simulink model "transistor_switch_1"  (Simulink 7.4)
settings: Solver=ode23s  StartTime=0.0  StopTime=200e-6  MaxStep=10e-9  RelTol=1e-4
libraries: powerlib x7, simpower_extensions_1 x1
settings Model: Creator=Dick  LastModifiedBy=Dick

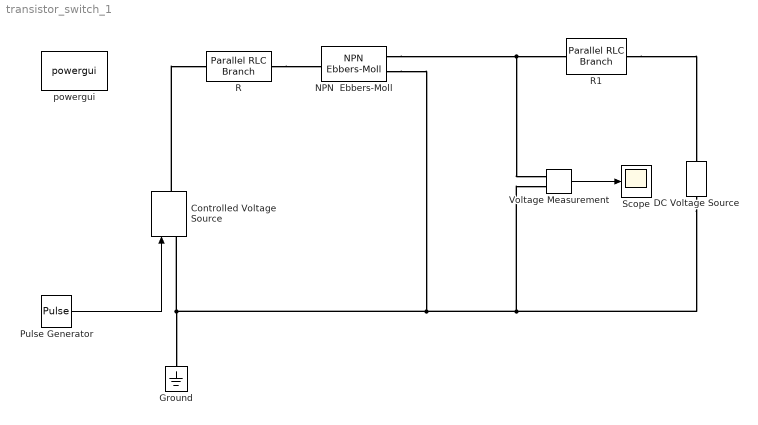
== system transistor_switch_1 ==
  " R" : powerlib/Elements/Parallel RLC Branch  DialogController=POWERSYS.PowerSysDialog  PhysicalDomain=powersysdomain  SubClassName=unknown  LeftPortType=p1  RightPortType=p1  LConnTagsString=a  RConnTagsString=__new0  BranchType=R  Resistance=1000  Inductance=1e-3  SetiL0=off  InitialCurrent=0  Capacitance=1e-6  Setx0=off  InitialVoltage=0  Measurements=None
  " R1" : powerlib/Elements/Parallel RLC Branch  DialogController=POWERSYS.PowerSysDialog  PhysicalDomain=powersysdomain  SubClassName=unknown  LeftPortType=p1  RightPortType=p1  LConnTagsString=a  RConnTagsString=__new0  BranchType=R  Resistance=100  Inductance=1e-3  SetiL0=off  InitialCurrent=0  Capacitance=1e-6  Setx0=off  InitialVoltage=0  Measurements=None
  Controlled Voltage Source : powerlib/Electrical Sources/Controlled Voltage Source  DialogController=POWERSYS.PowerSysDialog  SystemSampleTime=-1  Initialize=off  Source_Type=DC  Amplitude=0  Phase=0  Frequency=0  Measurements=None
  DC Voltage Source : powerlib/Electrical Sources/DC Voltage Source  DialogController=POWERSYS.PowerSysDialog  SystemSampleTime=-1  Amplitude=10  Measurements=None
  Ground : powerlib/Elements/Ground  DialogController=POWERSYS.PowerSysDialog  PhysicalDomain=powersysdomain  SubClassName=unknown  LeftPortType=p1  RightPortType=p1  LConnTagsString=a
  "NPN  Ebbers-Moll " : simpower_extensions_1/NPN  Ebbers-Moll   SystemSampleTime=-1  Beta=100  IEs=1e-12;  ICs=1e-12;  Ro=1e5  Cbc=5e-12  Cbe=100e-12  Rbb=100
  Pulse Generator : DiscretePulseGenerator  PulseType=Time based  Amplitude=5  Period=20e-6  PulseWidth=50  PhaseDelay=0  SampleTime=1
  Scope : Scope
      settings: YMin=-1  YMax=12  MaxDataPoints=500000
  Voltage Measurement : powerlib/Measurements/Voltage Measurement  DialogController=POWERSYS.PowerSysDialog  SystemSampleTime=-1  PhasorSimulation=off  OutputType=Complex  PSBequivalent=0
  powergui : powerlib/powergui  Priority=1  SystemSampleTime=-1  SimulationMode=Continuous  SampleTime=50e-6  frequency=60  SPID=off  DisableSnubberDevices=off  DisableRonSwitches=off  DisableVfSwitches=off  SwTol=0  Interpol=off  frequencyindice=0  echomessages=off  HookPort=off  DisplayEquations=off  FunctionMessages=off  EnableUseOfTLC=off  x0status=blocks  RestoreLinks=warning  Frange=[0:2:500]  Ylog=off  Xlog=on  ShowGrid=off  save=off  variable=ZData  ZoomFFT=on  StartTime=0.0  cycles=1  DisplayStyle=1  fundamental=60  FreqAxis=off  MaxFrequency=1000  frequencyindicesteady=1  RmsSteady=1  display=off  Ts=0  methode=off
  wires:
  Voltage Measurement/1 -> Scope/1
  Pulse Generator/1 -> Controlled Voltage Source/1
  connections:
  " R"/RConn1 -- "NPN  Ebbers-Moll "/LConn1
  "NPN  Ebbers-Moll "/RConn1 -- " R1"/LConn1 -- Voltage Measurement/LConn1
  Controlled Voltage Source/RConn1 -- " R"/LConn1
  "NPN  Ebbers-Moll "/RConn2 -- DC Voltage Source/LConn1 -- Voltage Measurement/LConn2 -- Controlled Voltage Source/LConn1 -- Ground/LConn1
  " R1"/RConn1 -- DC Voltage Source/RConn1
